simulink model "full_wave"  (R2024b)
settings: Solver=VariableStepAuto  StartTime=0.0  StopTime=10.0  RelTol=1e-3
values from neighbouring files (symbols this model uses):
  alpha_1_t = alpha_rad/(2*pi*f)    (= 0.00166666666667)    [simulink_params.m]
  alpha_2_t = alpha_2_rad/(2*pi*f)    (= 0.0116666666667)    [simulink_params.m]
  f = double(f)    [ChargeFWR.m]    (also in full_wave_rectifier_CT.m = @(xx) arrayfun(@(xval) compute_power_loss(xval, alpha, beta,; simulink_params.m = 50)
  R = 20    [simulink_params.m]
  Vin_peak = sqrt(2)*Vin_rms    [simulink_params.m]
libraries: spsThyristorLib x4, spsVoltageMeasurementLib x3, spsACVoltageSourceLib x1, spsCurrentMeasurementLib x1, spsMeanPhasorLib x1, spsSeriesRLCBranchLib x1, sps_lib x1
settings Model: Creator=George  LastModifiedBy=George

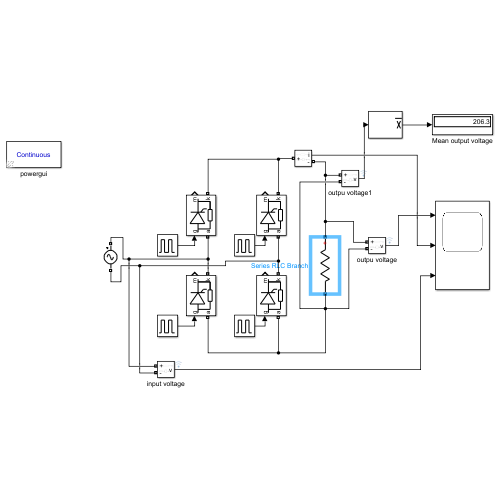
[thumbnail: Simulink's stored preview of the top-level diagram]
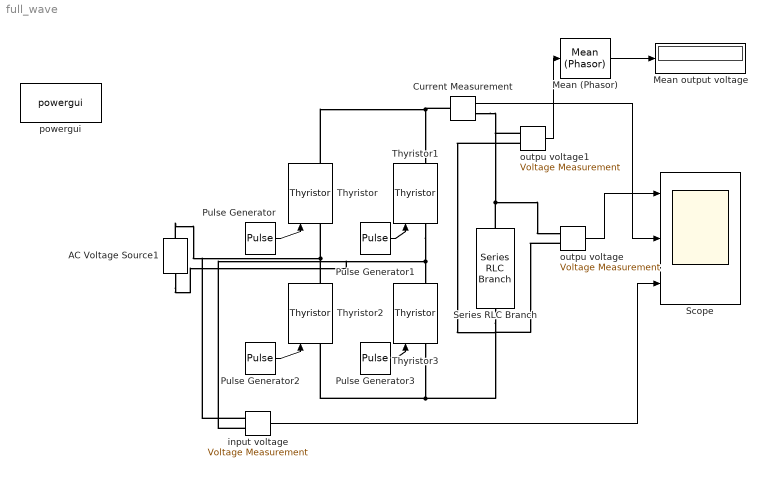
== system full_wave ==
  AC Voltage Source1 : spsACVoltageSourceLib/AC Voltage Source  Amplitude=Vin_peak  Phase=0  Frequency=f  SampleTime=0  Measurements=None  BusType=swing  Pref=10e3  Qref=0  Qmin=-inf  Qmax=+inf
  Current Measurement : spsCurrentMeasurementLib/Current Measurement  PhasorSimulation=off  OutputType=Complex  PSBequivalent=0
  Mean (Phasor) : spsMeanPhasorLib/Mean (Phasor)  Freq=60  Vinit=0  Ts=0
      settings: LibrarySourceBlock=|
      | sps_lib/Sensors and Measurements/Mean
      | (Phasor)
  Mean output voltage : Display
  Pulse Generator : DiscretePulseGenerator  PulseType=Time based  Amplitude=2  Period=1/f  PulseWidth=5  PhaseDelay=alpha_1_t
  Pulse Generator1 : DiscretePulseGenerator  PulseType=Time based  Amplitude=2  Period=1/f  PulseWidth=5  PhaseDelay=alpha_2_t
  Pulse Generator2 : DiscretePulseGenerator  PulseType=Time based  Amplitude=2  Period=1/f  PulseWidth=5  PhaseDelay=alpha_2_t
  Pulse Generator3 : DiscretePulseGenerator  PulseType=Time based  Amplitude=2  Period=1/f  PulseWidth=5  PhaseDelay=alpha_1_t
  Scope : Scope  NumInputPorts=3
  Series RLC Branch : spsSeriesRLCBranchLib/Series RLC Branch  LConnTagsString=__new0  RConnTagsString=__new0  BranchType=R  Resistance=R  Inductance=0.1  SetiL0=off  InitialCurrent=0  Capacitance=0  Setx0=off  InitialVoltage=0  Measurements=None
  Thyristor{,1..3} (4 alike) : spsThyristorLib/Thyristor  Ron=0.001  Lon=0  Vf=0.75  IC=0  Rs=500  Cs=250e-6  Measurements=on
  input voltage : spsVoltageMeasurementLib/Voltage Measurement  PhasorSimulation=off  OutputType=Complex  PSBequivalent=0
  outpu voltage : spsVoltageMeasurementLib/Voltage Measurement  PhasorSimulation=off  OutputType=Complex  PSBequivalent=0
  outpu voltage1 : spsVoltageMeasurementLib/Voltage Measurement  PhasorSimulation=off  OutputType=Complex  PSBequivalent=0
  powergui : sps_lib/powergui  Priority=1  SimulationMode=Continuous  SampleTime=50e-6  frequency=50  Iterations=50  frequencyindice=50  Pbase=100e6  ErrMax=1e-4  UnitsV=kV  UnitsW=MW  buscounter=0  FunctionMessages=off  echomessages=off  EnableUseOfTLC=off  CurrentSourceSwitches=off  DisableSnubberDevices=off  DisableRonSwitches=off  DisableVfSwitches=off  DisplayEquations=off  AutomaticDiscreteSolvers=off  SolverType=Tustin/Backward Euler (TBE)  Interpol=off  ExternalGateDelay=off  methode=off  Ts=100  x0status=blocks  SPID=on  SwTol=0  HookPort=off  NonlinearTolerance=1e-4  nMaxIteration=100  ContinueOnMaxIteration=off  RestoreLinks=warning  ResistiveCurrentMeasurement=off  Frange=[0:2:500]  Ylog=off  Xlog=on  ShowGrid=off  save=off  variable=ZData  structure=0  ZoomFFT=off  StartTime=0.0  cycles=1  DisplayStyle=1  fundamental=60  FreqAxis=off  MaxFrequency=1000  frequencyindicesteady=1  RmsSteady=1  display=off
  wires:
  Mean (Phasor)/1 -> Mean output voltage/1
  Pulse Generator/1 -> Thyristor/1
  Pulse Generator1/1 -> Thyristor1/1
  Pulse Generator3/1 -> Thyristor3/1
  Pulse Generator2/1 -> Thyristor2/1
  input voltage/1 -> Scope/3
  Current Measurement/1 -> Scope/2
  outpu voltage1/1 -> Mean (Phasor)/1
  outpu voltage/1 -> Scope/1
  connections:
  Thyristor2/RConn1 -- input voltage/LConn1 -- AC Voltage Source1/RConn1 -- Thyristor/LConn1
  Thyristor3/LConn1 -- outpu voltage1/LConn2 -- outpu voltage/LConn2 -- Series RLC Branch/RConn1 -- Thyristor2/LConn1
  Thyristor1/LConn1 -- input voltage/LConn2 -- AC Voltage Source1/LConn1 -- Thyristor3/RConn1
  Series RLC Branch/LConn1 -- outpu voltage1/LConn1 -- Current Measurement/RConn1 -- outpu voltage/LConn1
  Thyristor/RConn1 -- Current Measurement/LConn1 -- Thyristor1/RConn1
